simulink model "P06"  (R2023a)
settings: Solver=VariableStepAuto  StartTime=0.0  StopTime=10.0  RelTol=1e-3
settings Model: Creator=tgz8009  LastModifiedBy=tgz8009

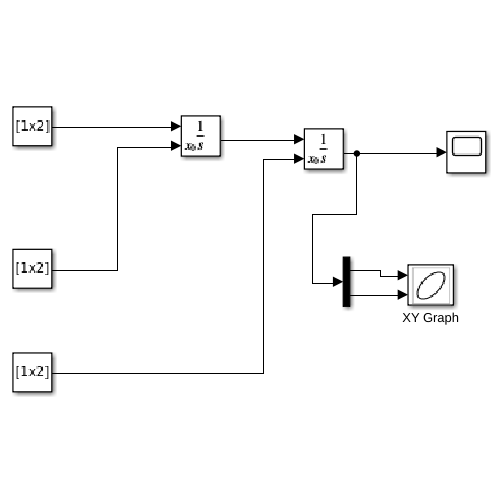
[thumbnail: Simulink's stored preview of the top-level diagram]
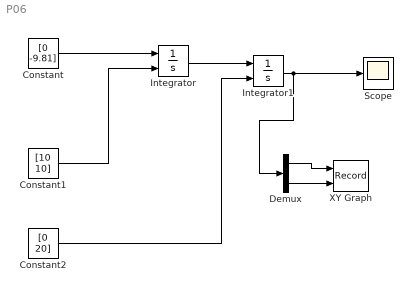
== system P06 ==
  Constant : Constant  Value=[0 -9.81]
  Constant1 : Constant  Value=[10 10]
  Constant2 : Constant  Value=[0 20]
  Demux : Demux  Outputs=2
  Integrator : Integrator  InitialConditionSource=external
  Integrator1 : Integrator  InitialConditionSource=external
  Scope : Scope
  XY Graph : Record  FileSettingsInternal="{\"entries\":[{\"content\":{\"excelSettings\":{\"content\":{},\"type\":\"Streamout.ExcelSettings\"}},\"type\":\"Streamout.FileSettingStorage\",\"uuid\":\"bb0139dd-d603-4d15-a757-0d48beffa6b3\"}],\"packageUris\":[\"http://schema.mathworks.com/mf0/streamout_blocks/R2020a\"],\"version\":\"1.0\"}"  Layout=[1 1]  SignalsInternal="{\"entries\":[{\"content\":{\"signals\":[{\"content\":{\"blockPath\":[\"untitled/XY Graph\"],\"dimensions\":[1],\"domain\":\"untitled/XY Graph\",\"lineColor\":\"#a2142f\",\"plots\":[1],\"port\":1,\"sid\":[\"\"],\"signalID\":27},\"type\":\"RecordBlkView.Signal\",\"uuid\":\"3859e4c2-2333-4ef4-ab33-6c9bd675c695\"},{\"content\":{\"blockPath\":[\"untitled/XY Graph\"],\"dimensions\":[1],\"domain\":\"untitled/XY Graph\",\"lineColor\":\"#139fff\",\"plots\":[1],\"port\":2,\"sid\":[\"\"],\"signalID\":31},\"type\":\"RecordBlkView.Signal\",\"uuid\":\"33811210-1635-4038-ad19-848bf2a004c6\"}]},\"type\":\"RecordBlkView.InputSignals\",\"uuid\":\"635063ec-de12-4611-8516-94f7ca20c2f9\"}],\"packageUris\":[\"http://schema.mathworks.com/mf0/streamout_blocks/R2020a\"],\"version\":\"1.0\"}"  VisualizationBindings="{\"xyplotplugin\":{\"info\":[{\"series\":[{\"bindingParametersList\":[{\"parameter\":\"X-Axis\",\"signalID\":27,\"signalName\":\"XY Graph:1\"},{\"parameter\":\"Y-Axis\",\"signalID\":31,\"signalName\":\"XY Graph:2\"}],\"seriesID\":10108}],\"subplotID\":1}]}}"  CompatibilityTag=XY
  wires:
  Constant/1 -> Integrator/1
  Integrator/1 -> Integrator1/1
  Constant2/1 -> Integrator1/2
  Constant1/1 -> Integrator/2
  Integrator1/1 -> Demux/1, Scope/1
  Demux/2 -> XY Graph/2
  Demux/1 -> XY Graph/1
